simulink model "mds_accelerometer"  (Simulink 7.7)
settings: Solver=ode45  StartTime=0.0  StopTime=400  RelTol=1e-3
settings Model: Creator=Rohan  LastModifiedBy=Rohan

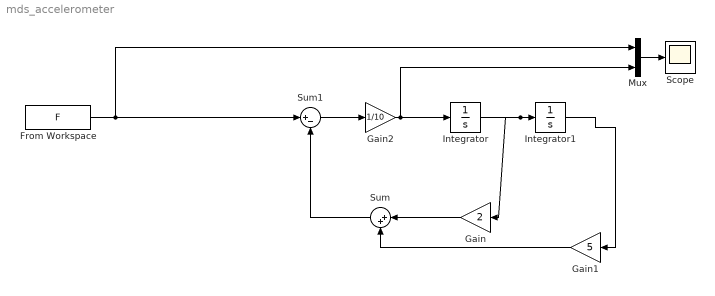
== system mds_accelerometer ==
  From Workspace : FromWorkspace  VariableName=F  SampleTime=0
  Gain : Gain  Gain=2
  Gain1 : Gain  Gain=5
  Gain2 : Gain  Gain=1/10
  Integrator : Integrator
  Integrator1 : Integrator
  Mux : Mux  Inputs=2
  Scope : Scope
      settings: TimeRange=100  YMin=-0.2  YMax=1.2
  Sum : Sum  Inputs=|++
  Sum1 : Sum  Inputs=|+-
  wires:
  Integrator/1 -> Integrator1/1, Gain/1
  Integrator1/1 -> Gain1/1
  Gain2/1 -> Integrator/1, Mux/2
  Gain/1 -> Sum/1
  Gain1/1 -> Sum/2
  Sum1/1 -> Gain2/1
  Sum/1 -> Sum1/2
  Mux/1 -> Scope/1
  From Workspace/1 -> Sum1/1, Mux/1
